simulink model "DNN_x3D_M_2000iA900L_with_6_rev"  (R2022a)
settings: Solver=VariableStepAuto  StartTime=0.0  StopTime=10.0  RelTol=1e-3
model workspace: external: MATLAB File /home/archistrax/Desktop/DNN/Simulink/Brazo robotico (2)/x3D_M_2000iA900L_OLGA_DataFile8.m (data not in the file)
values from neighbouring files (symbols this model uses):
  smiData = struct    [x3D_M_2000iA900L_OLGA_DataFile8.m]
undefined symbols (not defined in the file or in its folder): X, Y, Z
libraries: sm_lib x78, nesl_utility x31, slpidlib x15, matrix_library x4
(part 4 of 4)

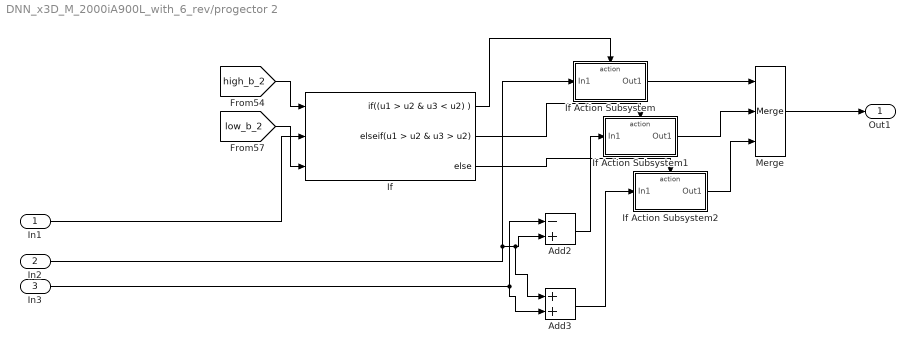
== system DNN_x3D_M_2000iA900L_with_6_rev/progector 2 ==
  In1 : Inport
  In2 : Inport  Port=2
  In3 : Inport  Port=3
  Add2 : Sum  Inputs=-+
  Add3 : Sum
  If : If  NumInputs=3  IfExpression=(u1 > u2 & u3 < u2)  ElseIfExpressions=u1 > u2 & u3 > u2
  If Action Subsystem : Subsystem  TreatAsAtomicUnit=on
  If Action Subsystem1 : Subsystem  TreatAsAtomicUnit=on
  If Action Subsystem2 : Subsystem  TreatAsAtomicUnit=on
  Merge : Merge  Inputs=3
  Out1 : Outport
  wires:
  In1/1 -> If/2
  In3/1 -> Add3/2, Add2/1
  In2/1 -> If Action Subsystem/1(In1), Add3/1, Add2/2
  If/1 -> If Action Subsystem/Action
  Add3/1 -> If Action Subsystem2/1(In1)
  If Action Subsystem/1(Out1) -> Merge/1
  If/2 -> If Action Subsystem1/Action
  If Action Subsystem1/1(Out1) -> Merge/2
  If Action Subsystem2/1(Out1) -> Merge/3
  If/3 -> If Action Subsystem2/Action
  Add2/1 -> If Action Subsystem1/1(In1)
  Merge/1 -> Out1/1
  [high_b_2] -> If/1
  [low_b_2] -> If/3

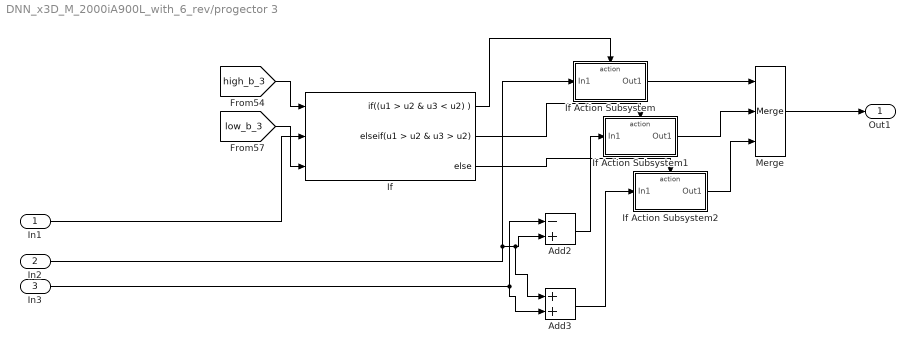
== system DNN_x3D_M_2000iA900L_with_6_rev/progector 3 ==
  In1 : Inport
  In2 : Inport  Port=2
  In3 : Inport  Port=3
  Add2 : Sum  Inputs=-+
  Add3 : Sum
  If : If  NumInputs=3  IfExpression=(u1 > u2 & u3 < u2)  ElseIfExpressions=u1 > u2 & u3 > u2
  If Action Subsystem : Subsystem  TreatAsAtomicUnit=on
  If Action Subsystem1 : Subsystem  TreatAsAtomicUnit=on
  If Action Subsystem2 : Subsystem  TreatAsAtomicUnit=on
  Merge : Merge  Inputs=3
  Out1 : Outport
  wires:
  In1/1 -> If/2
  In3/1 -> Add3/2, Add2/1
  In2/1 -> If Action Subsystem/1(In1), Add3/1, Add2/2
  If/1 -> If Action Subsystem/Action
  Add3/1 -> If Action Subsystem2/1(In1)
  If Action Subsystem/1(Out1) -> Merge/1
  If/2 -> If Action Subsystem1/Action
  If Action Subsystem1/1(Out1) -> Merge/2
  If Action Subsystem2/1(Out1) -> Merge/3
  If/3 -> If Action Subsystem2/Action
  Add2/1 -> If Action Subsystem1/1(In1)
  Merge/1 -> Out1/1
  [high_b_3] -> If/1
  [low_b_3] -> If/3

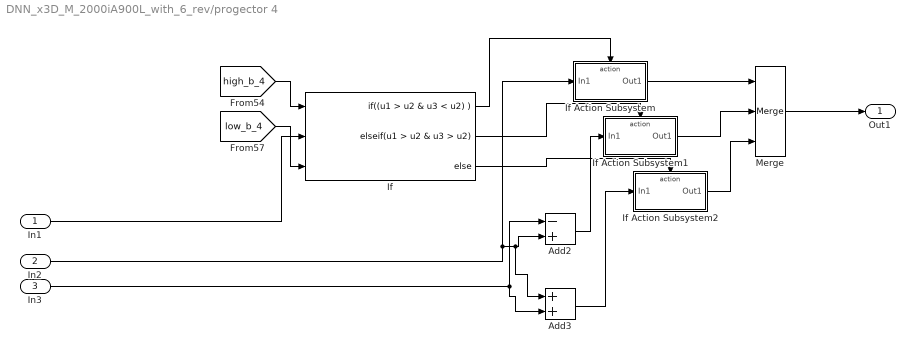
== system DNN_x3D_M_2000iA900L_with_6_rev/progector 4 ==
  In1 : Inport
  In2 : Inport  Port=2
  In3 : Inport  Port=3
  Add2 : Sum  Inputs=-+
  Add3 : Sum
  If : If  NumInputs=3  IfExpression=(u1 > u2 & u3 < u2)  ElseIfExpressions=u1 > u2 & u3 > u2
  If Action Subsystem : Subsystem  TreatAsAtomicUnit=on
  If Action Subsystem1 : Subsystem  TreatAsAtomicUnit=on
  If Action Subsystem2 : Subsystem  TreatAsAtomicUnit=on
  Merge : Merge  Inputs=3
  Out1 : Outport
  wires:
  In1/1 -> If/2
  In3/1 -> Add3/2, Add2/1
  In2/1 -> If Action Subsystem/1(In1), Add3/1, Add2/2
  If/1 -> If Action Subsystem/Action
  Add3/1 -> If Action Subsystem2/1(In1)
  If Action Subsystem/1(Out1) -> Merge/1
  If/2 -> If Action Subsystem1/Action
  If Action Subsystem1/1(Out1) -> Merge/2
  If Action Subsystem2/1(Out1) -> Merge/3
  If/3 -> If Action Subsystem2/Action
  Add2/1 -> If Action Subsystem1/1(In1)
  Merge/1 -> Out1/1
  [high_b_4] -> If/1
  [low_b_4] -> If/3

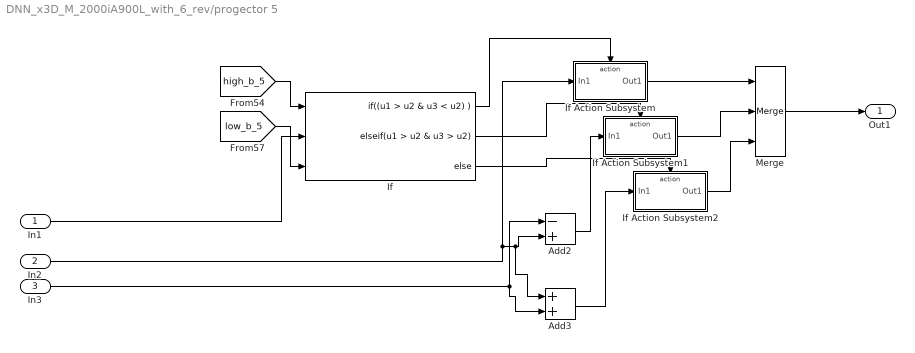
== system DNN_x3D_M_2000iA900L_with_6_rev/progector 5 ==
  In1 : Inport
  In2 : Inport  Port=2
  In3 : Inport  Port=3
  Add2 : Sum  Inputs=-+
  Add3 : Sum
  If : If  NumInputs=3  IfExpression=(u1 > u2 & u3 < u2)  ElseIfExpressions=u1 > u2 & u3 > u2
  If Action Subsystem : Subsystem  TreatAsAtomicUnit=on
  If Action Subsystem1 : Subsystem  TreatAsAtomicUnit=on
  If Action Subsystem2 : Subsystem  TreatAsAtomicUnit=on
  Merge : Merge  Inputs=3
  Out1 : Outport
  wires:
  In1/1 -> If/2
  In3/1 -> Add3/2, Add2/1
  In2/1 -> If Action Subsystem/1(In1), Add3/1, Add2/2
  If/1 -> If Action Subsystem/Action
  Add3/1 -> If Action Subsystem2/1(In1)
  If Action Subsystem/1(Out1) -> Merge/1
  If/2 -> If Action Subsystem1/Action
  If Action Subsystem1/1(Out1) -> Merge/2
  If Action Subsystem2/1(Out1) -> Merge/3
  If/3 -> If Action Subsystem2/Action
  Add2/1 -> If Action Subsystem1/1(In1)
  Merge/1 -> Out1/1
  [high_b_5] -> If/1
  [low_b_5] -> If/3

== system DNN_x3D_M_2000iA900L_with_6_rev/progector 6 ==
  In1 : Inport
  In2 : Inport  Port=2
  In3 : Inport  Port=3
  Add2 : Sum  Inputs=-+
  Add3 : Sum
  If : If  NumInputs=3  IfExpression=(u1 > u2 & u3 < u2)  ElseIfExpressions=u1 > u2 & u3 > u2
  If Action Subsystem : Subsystem  TreatAsAtomicUnit=on
  If Action Subsystem1 : Subsystem  TreatAsAtomicUnit=on
  If Action Subsystem2 : Subsystem  TreatAsAtomicUnit=on
  Merge : Merge  Inputs=3
  Out1 : Outport
  wires:
  In1/1 -> If/2
  In3/1 -> Add3/2, Add2/1
  In2/1 -> If Action Subsystem/1(In1), Add3/1, Add2/2
  If/1 -> If Action Subsystem/Action
  Add3/1 -> If Action Subsystem2/1(In1)
  If Action Subsystem/1(Out1) -> Merge/1
  If/2 -> If Action Subsystem1/Action
  If Action Subsystem1/1(Out1) -> Merge/2
  If Action Subsystem2/1(Out1) -> Merge/3
  If/3 -> If Action Subsystem2/Action
  Add2/1 -> If Action Subsystem1/1(In1)
  Merge/1 -> Out1/1
  [high_b_6] -> If/1
  [low_b_6] -> If/3

== system DNN_x3D_M_2000iA900L_with_6_rev/projector 1 ==
  In1 : Inport
  In2 : Inport  Port=2
  In3 : Inport  Port=3
  Add2 : Sum  Inputs=-+
  Add3 : Sum
  If : If  NumInputs=3  IfExpression=(u1 > u2 & u3 < u2)  ElseIfExpressions=u1 > u2 & u3 > u2
  If Action Subsystem : Subsystem  TreatAsAtomicUnit=on
  If Action Subsystem1 : Subsystem  TreatAsAtomicUnit=on
  If Action Subsystem2 : Subsystem  TreatAsAtomicUnit=on
  Merge : Merge  Inputs=3
  Out1 : Outport
  wires:
  In1/1 -> If/2
  In3/1 -> Add3/2, Add2/1
  In2/1 -> If Action Subsystem/1(In1), Add3/1, Add2/2
  If/1 -> If Action Subsystem/Action
  Add3/1 -> If Action Subsystem2/1(In1)
  If Action Subsystem/1(Out1) -> Merge/1
  If/2 -> If Action Subsystem1/Action
  If Action Subsystem1/1(Out1) -> Merge/2
  If Action Subsystem2/1(Out1) -> Merge/3
  If/3 -> If Action Subsystem2/Action
  Add2/1 -> If Action Subsystem1/1(In1)
  Merge/1 -> Out1/1
  [high_b_1] -> If/1
  [low_b_1] -> If/3

== system DNN_x3D_M_2000iA900L_with_6_rev/progector 2/If Action Subsystem ==
  In1 : Inport
  Action Port : ActionPort  ActionPortLabel=if((u1 > u2 & u3 < u2) )
  Out1 : Outport
  wires:
  In1/1 -> Out1/1

== system DNN_x3D_M_2000iA900L_with_6_rev/progector 2/If Action Subsystem1 ==
  In1 : Inport
  Action Port : ActionPort  ActionPortLabel=elseif(u1 > u2 & u3 > u2)
  Out1 : Outport
  wires:
  In1/1 -> Out1/1

== system DNN_x3D_M_2000iA900L_with_6_rev/progector 2/If Action Subsystem2 ==
  In1 : Inport
  Action Port : ActionPort  ActionPortLabel=else
  Out1 : Outport
  wires:
  In1/1 -> Out1/1

== system DNN_x3D_M_2000iA900L_with_6_rev/progector 3/If Action Subsystem ==
  In1 : Inport
  Action Port : ActionPort  ActionPortLabel=if((u1 > u2 & u3 < u2) )
  Out1 : Outport
  wires:
  In1/1 -> Out1/1

== system DNN_x3D_M_2000iA900L_with_6_rev/progector 3/If Action Subsystem1 ==
  In1 : Inport
  Action Port : ActionPort  ActionPortLabel=elseif(u1 > u2 & u3 > u2)
  Out1 : Outport
  wires:
  In1/1 -> Out1/1

== system DNN_x3D_M_2000iA900L_with_6_rev/progector 3/If Action Subsystem2 ==
  In1 : Inport
  Action Port : ActionPort  ActionPortLabel=else
  Out1 : Outport
  wires:
  In1/1 -> Out1/1

== system DNN_x3D_M_2000iA900L_with_6_rev/progector 4/If Action Subsystem ==
  In1 : Inport
  Action Port : ActionPort  ActionPortLabel=if((u1 > u2 & u3 < u2) )
  Out1 : Outport
  wires:
  In1/1 -> Out1/1

== system DNN_x3D_M_2000iA900L_with_6_rev/progector 4/If Action Subsystem1 ==
  In1 : Inport
  Action Port : ActionPort  ActionPortLabel=elseif(u1 > u2 & u3 > u2)
  Out1 : Outport
  wires:
  In1/1 -> Out1/1

== system DNN_x3D_M_2000iA900L_with_6_rev/progector 4/If Action Subsystem2 ==
  In1 : Inport
  Action Port : ActionPort  ActionPortLabel=else
  Out1 : Outport
  wires:
  In1/1 -> Out1/1

== system DNN_x3D_M_2000iA900L_with_6_rev/progector 5/If Action Subsystem ==
  In1 : Inport
  Action Port : ActionPort  ActionPortLabel=if((u1 > u2 & u3 < u2) )
  Out1 : Outport
  wires:
  In1/1 -> Out1/1

== system DNN_x3D_M_2000iA900L_with_6_rev/progector 5/If Action Subsystem1 ==
  In1 : Inport
  Action Port : ActionPort  ActionPortLabel=elseif(u1 > u2 & u3 > u2)
  Out1 : Outport
  wires:
  In1/1 -> Out1/1

== system DNN_x3D_M_2000iA900L_with_6_rev/progector 5/If Action Subsystem2 ==
  In1 : Inport
  Action Port : ActionPort  ActionPortLabel=else
  Out1 : Outport
  wires:
  In1/1 -> Out1/1

== system DNN_x3D_M_2000iA900L_with_6_rev/progector 6/If Action Subsystem ==
  In1 : Inport
  Action Port : ActionPort  ActionPortLabel=if((u1 > u2 & u3 < u2) )
  Out1 : Outport
  wires:
  In1/1 -> Out1/1

== system DNN_x3D_M_2000iA900L_with_6_rev/progector 6/If Action Subsystem1 ==
  In1 : Inport
  Action Port : ActionPort  ActionPortLabel=elseif(u1 > u2 & u3 > u2)
  Out1 : Outport
  wires:
  In1/1 -> Out1/1

== system DNN_x3D_M_2000iA900L_with_6_rev/progector 6/If Action Subsystem2 ==
  In1 : Inport
  Action Port : ActionPort  ActionPortLabel=else
  Out1 : Outport
  wires:
  In1/1 -> Out1/1

== system DNN_x3D_M_2000iA900L_with_6_rev/projector 1/If Action Subsystem ==
  In1 : Inport
  Action Port : ActionPort  ActionPortLabel=if((u1 > u2 & u3 < u2) )
  Out1 : Outport
  wires:
  In1/1 -> Out1/1

== system DNN_x3D_M_2000iA900L_with_6_rev/projector 1/If Action Subsystem1 ==
  In1 : Inport
  Action Port : ActionPort  ActionPortLabel=elseif(u1 > u2 & u3 > u2)
  Out1 : Outport
  wires:
  In1/1 -> Out1/1

== system DNN_x3D_M_2000iA900L_with_6_rev/projector 1/If Action Subsystem2 ==
  In1 : Inport
  Action Port : ActionPort  ActionPortLabel=else
  Out1 : Outport
  wires:
  In1/1 -> Out1/1
